simulink model "Bai_7"  (R2020b)
settings: Solver=VariableStepAuto  StartTime=0.0  StopTime=10.0  RelTol=1e-3
undefined symbols (not defined in the file): F
settings Model: Creator=John Andrew  LastModifiedBy=John Andrew

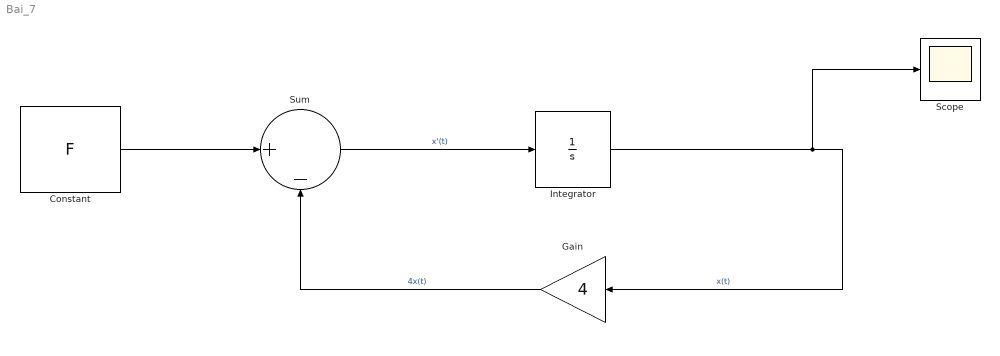
== system Bai_7 ==
  Constant : Constant  Value=F
  Gain : Gain  Gain=4
  Integrator : Integrator
  Scope : Scope
  Sum : Sum  Inputs=|+-
  wires:
  Sum/1 -> Integrator/1  "x'(t)"
  Gain/1 -> Sum/2  "4x(t)"
  Constant/1 -> Sum/1
  Integrator/1 -> Scope/1, Gain/1  "x(t)"
